simulink model "TopLevel_Throttle"  (R2019b)
settings: Solver=VariableStepAuto  StartTime=0.0  StopTime=10.0  FixedStep=0.1  RelTol=1e-3
undefined symbols (not defined in the file): sigbuilder_block
settings Model: Creator=spuny  LastModifiedBy=spuny

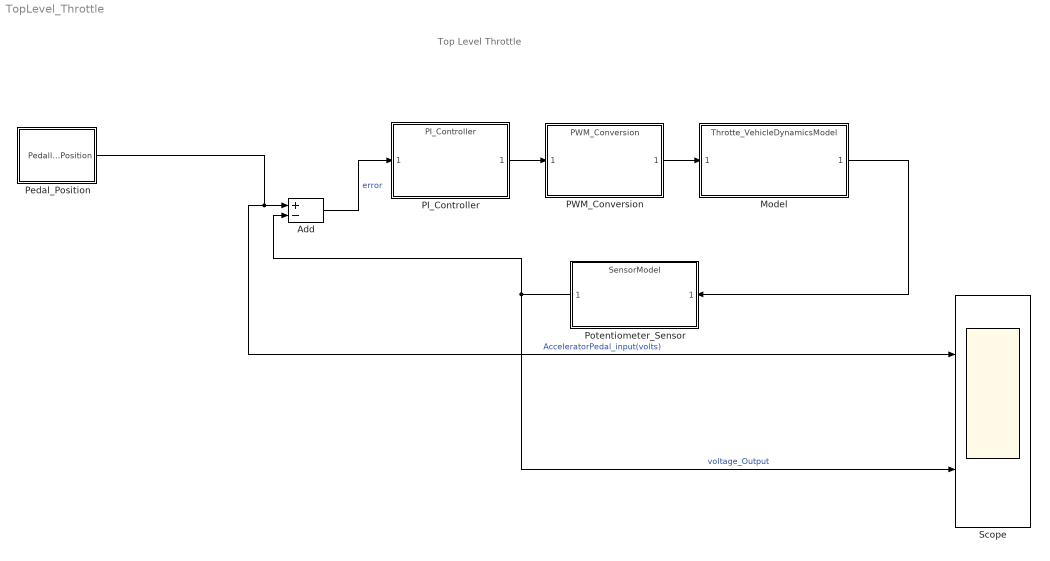
== system TopLevel_Throttle ==
  note: Top Level Throttle
  Add : Sum  Inputs=+-
  Model : ModelReference  ModelNameDialog=Throtte_VehicleDynamicsModel.slx  SimulationMode=Normal  ModelReferenceVersion=1.19
  PI_Controller : ModelReference  ModelNameDialog=PI_Controller.slx  SimulationMode=Normal  ModelReferenceVersion=1.5
  PWM_Conversion : ModelReference  ModelNameDialog=PWM_Conversion.slx  SimulationMode=Normal  ModelReferenceVersion=1.5
  Pedal_Position : Subsystem
  "Potentiometer_Sensor " : ModelReference  ModelNameDialog=SensorModel.slx  SimulationMode=Normal  ModelReferenceVersion=1.12
  Scope : Scope  NumInputPorts=2
  wires:
  PI_Controller/1 -> PWM_Conversion/1
  Add/1 -> PI_Controller/1  "error"
  "Potentiometer_Sensor "/1 -> Add/2, Scope/2  "voltage_Output"
  Pedal_Position/1(Pedall_Position) -> Scope/1, Add/1  "AcceleratorPedal_input(volts)"
  PWM_Conversion/1 -> Model/1
  Model/1 -> "Potentiometer_Sensor "/1

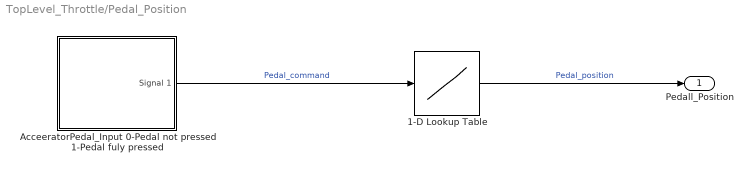
== system TopLevel_Throttle/Pedal_Position ==
  1-D Lookup Table : Lookup_n-D  NumberOfTableDimensions=1  BreakpointsForDimension1=[0 1]  Table=[0.5 4.5]  ExtrapMethod=Clip  InternalRulePriority=Speed  RndMeth=Simplest  InputSameDT=on
  "AcceeratorPedal_Input 0-Pedal not pressed 1-Pedal fuly pressed " : Subsystem  Tag=STV Subsys  LoadFcn=sigbuilder_block('load');  StartFcn=sigbuilder_block('start');  StopFcn=sigbuilder_block('stop');  ClipboardFcn=sigbuilder_block('clipboard');  mask(Sigbuilder block){tuvar=[0:10]}
      mask help: Simulink:masks:SigbuilderBlock_MD
      mask init:
      | if ~strcmp(get_param(bdroot(gcbh),'SimulationStatus'),'stopped') tuvar = sigbuilder_block('maskInit'); end
      settings: CopyFcn=sigbuilder_block('copy');  DeleteFcn=sigbuilder_block('delete');  ModelCloseFcn=sigbuilder_block('modelClose');  PreSaveFcn=sigbuilder_block('preSave');  PauseFcn=sigbuilder_block('pause');  ContinueFcn=sigbuilder_block('continue');  NameChangeFcn=sigbuilder_block('namechange');  OpenFcn=sigbuilder_block('open',[318.75 130.5 550.5 331.5 ]);  CloseFcn=sigbuilder_block('close');
      mask Display: plot(0, 0, 100, 100,[2, 2, 32, 32, 2], [68, 8, 8, 68, 68],[32, 2], [38, 38], [32, 19, 2],[53, 60, 44], [32, 17, 17, 2],[16, 16, 31, 31]);txt = getActiveGroup(gcbh);text(2, 100, txt,'verticalAlignment', 'top');
  Pedall_Position : Outport
  wires:
  "AcceeratorPedal_Input 0-Pedal not pressed 1-Pedal fuly pressed "/1(Signal 1) -> 1-D Lookup Table/1  "Pedal_command"
  1-D Lookup Table/1 -> Pedall_Position/1  "Pedal_position"

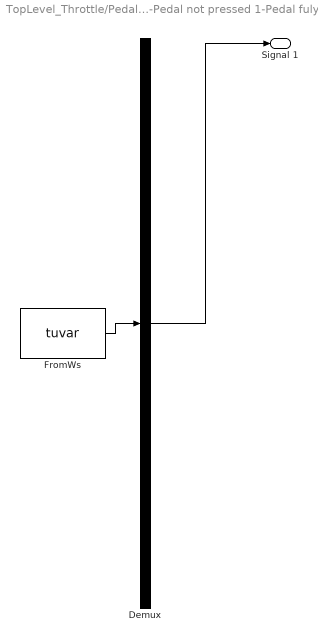
== system TopLevel_Throttle/Pedal_Position/AcceeratorPedal_Input 0-Pedal not pressed 1-Pedal fuly pressed  ==
  Demux : Demux  Tag=STV Demux  Outputs=1
  FromWs : FromWorkspace  Tag=STV FromWs  VariableName=tuvar  SampleTime=0
      SigBuilderData=|
      | common.afterFinalStr = 'Extrapolate'
      | common.sampleTime = 0
      | dataSet.timeRange = [0 10]
      | dataSet.name = 'Group 1'
      | sbobj.Groups.Name = 'Group 1'
      | sbobj.Groups.Signals.Name = 'Signal 1'
      | sbobj.Groups.Signals.XData = [0 4 4 6 6 10]
      | sbobj.Groups.Signals.YData = [-0.05 0.195 0.505 0.645 0.095 -0.09]
  Signal 1 : Outport  Tag=STV Outport
  wires:
  Demux/1 -> Signal 1/1
  FromWs/1 -> Demux/1
